simulink model "Mux_Demux2"  (R2017b)
settings: Solver=FixedStepDiscrete  StartTime=0.0  StopTime=10.0  FixedStep=0.200000  RelTol=1e-3
undefined symbols (not defined in the file): a, b
settings Model: Creator=hbourbou  LastModifiedBy=hbourbou
settings DataIOCC: SaveFormat=StructureWithTime
settings OptimizationCC: LifeSpan=inf
settings DebuggingCC: SFExecutionAtInitializationDiag=none
settings HardwareCC: ProdBitPerSizeT=32  ProdBitPerPtrDiffT=32  ProdWordSize=32  ProdHWDeviceType=Specified
settings CodeAppCC: StateflowObjectComments=on

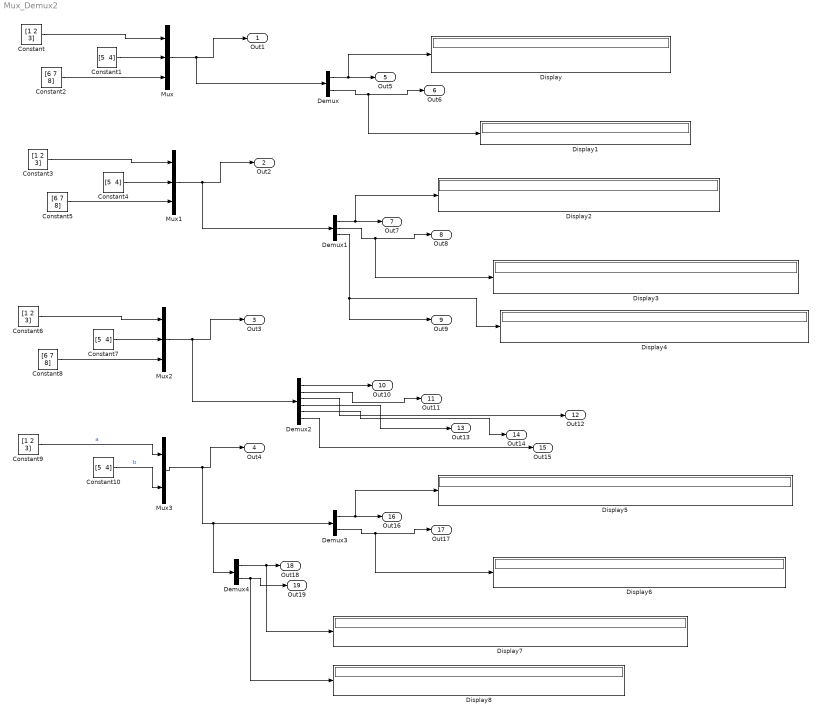
== system Mux_Demux2 ==
  Constant : Constant  Value=[1 2 3]
  Constant1 : Constant  Value="[5  4]"
  Constant10 : Constant  Value="[5  4]"
  Constant2 : Constant  Value=[6 7 8]
  Constant3 : Constant  Value=[1 2 3]  OutDataTypeStr=int8
  Constant4 : Constant  Value="[5  4]"  OutDataTypeStr=int8
  Constant5 : Constant  Value=[6 7 8]  OutDataTypeStr=int8
  Constant6 : Constant  Value=[1 2 3]
  Constant7 : Constant  Value="[5  4]"
  Constant8 : Constant  Value=[6 7 8]
  Constant9 : Constant  Value=[1 2 3]
  Demux : Demux  Outputs=2
  Demux1 : Demux  Outputs=3
  Demux2 : Demux  Outputs=6
  Demux3 : Demux  Outputs=[2 3]
  Demux4 : Demux  Outputs=2
  Display{,1..8} (9 alike) : Display
  Mux : Mux  Inputs=3
  Mux1 : Mux  Inputs=[3,2,3]
  Mux2 : Mux  Inputs={3,2,3}
  Mux3 : Mux  Inputs=a,b
  Out1 : Outport
  Out2 : Outport  Port=2
  Out3 : Outport  Port=3
  Out4 : Outport  Port=4
  Out5 : Outport  Port=5
  Out6 : Outport  Port=6
  Out7 : Outport  Port=7
  Out8 : Outport  Port=8
  Out9 : Outport  Port=9
  Out10 : Outport  Port=10
  Out11 : Outport  Port=11
  Out12 : Outport  Port=12
  Out13 : Outport  Port=13
  Out14 : Outport  Port=14
  Out15 : Outport  Port=15
  Out16 : Outport  Port=16
  Out17 : Outport  Port=17
  Out18 : Outport  Port=18
  Out19 : Outport  Port=19
  wires:
  Mux/1 -> Demux/1, Out1/1
  Constant2/1 -> Mux/3
  Constant1/1 -> Mux/2
  Constant/1 -> Mux/1
  Constant5/1 -> Mux1/3
  Constant4/1 -> Mux1/2
  Constant3/1 -> Mux1/1
  Constant8/1 -> Mux2/3
  Constant7/1 -> Mux2/2
  Constant6/1 -> Mux2/1
  Constant10/1 -> Mux3/2  "b"
  Constant9/1 -> Mux3/1  "a"
  Demux/1 -> Display/1, Out5/1
  Demux/2 -> Display1/1, Out6/1
  Mux1/1 -> Demux1/1, Out2/1
  Demux1/1 -> Display2/1, Out7/1
  Demux1/2 -> Display3/1, Out8/1
  Demux1/3 -> Display4/1, Out9/1
  Mux2/1 -> Demux2/1, Out3/1
  Demux2/1 -> Out10/1
  Demux2/2 -> Out11/1
  Demux2/3 -> Out12/1
  Demux2/4 -> Out13/1
  Demux2/5 -> Out14/1
  Demux2/6 -> Out15/1
  Mux3/1 -> Demux4/1, Demux3/1, Out4/1
  Demux3/1 -> Display5/1, Out16/1
  Demux3/2 -> Display6/1, Out17/1
  Demux4/1 -> Display7/1, Out18/1
  Demux4/2 -> Display8/1, Out19/1
